simulink subsystem "PvtSubSys_LSM"  (R2020b)
settings: Solver=VariableStepAuto  StartTime=0.0  StopTime=10.0  RelTol=1e-3
values from neighbouring files (symbols this model uses):
  P_LSM_ALC_Enable = 0.0    [LSM_Parameter.sldd]
  P_LSM_DOP_C0_EN_Limit = 0.8    [LSM_Parameter.sldd]
  P_LSM_DOP_C0_out_Limit = 2.0    [LSM_Parameter.sldd]
  P_LSM_DOP_C1_EN_Limit : value not decoded    [LSM_Parameter.sldd]
  P_LSM_DOP_C1_out_Limit : value not decoded    [LSM_Parameter.sldd]
  P_LSM_DOP_C1AndC2_Lim_X : value not decoded    [LSM_Parameter.sldd]
  P_LSM_DOP_C2_EN_Limit : value not decoded    [LSM_Parameter.sldd]
  P_LSM_DOP_C2_out_Limit : value not decoded    [LSM_Parameter.sldd]
  P_LSM_DOP_In_Pre2Dop_Dis = 1.0    [LSM_Parameter.sldd]
  P_LSM_DOP_Out_Pre2Dop_Dis = 2.0    [LSM_Parameter.sldd]
  P_LSM_DOP_PreDis_X : value not decoded    [LSM_Parameter.sldd]
  P_LSM_DOP_PreDis_Y : value not decoded    [LSM_Parameter.sldd]
  P_LSM_DOPValid_CheckTime = 0.06    [LSM_Parameter.sldd]
  P_LSM_DoubleLine_Curr2Cent_Dislimit = 0.5    [LSM_Parameter.sldd]
  P_LSM_DoubleLine_Dop2Cent_Dislimit = 0.5    [LSM_Parameter.sldd]
  P_LSM_DoubleLine_DOPOut_C1 : value not decoded    [LSM_Parameter.sldd]
  P_LSM_DoubleLine_Pre2Cent_Dislimit = 1.0    [LSM_Parameter.sldd]
  P_LSM_IFV2CenterAxis = 0.0    [LSM_Parameter.sldd]
  P_LSM_IFV2RearAxis = 0.0    [LSM_Parameter.sldd]
  P_LSM_LineSTD_Limit = 0.15    [LSM_Parameter.sldd]
  P_LSM_NOH_Switch = 0.0    [LSM_Parameter.sldd]
  P_LSM_Pre_t = 0.0    [LSM_Parameter.sldd]
  P_LSM_SingleLine_Cent2Edge_Dislimit = 100.0    [LSM_Parameter.sldd]
  P_LSM_SingleLine_Curr2Cent_Dislimit = 0.2    [LSM_Parameter.sldd]
  P_LSM_SingleLine_Dop2Cent_Dislimit = 0.2    [LSM_Parameter.sldd]
  P_LSM_SingleLine_DOPOut_C1 : value not decoded    [LSM_Parameter.sldd]
  P_LSM_SingleLine_Pre2Cent_Dislimit = 0.5    [LSM_Parameter.sldd]
undefined symbols (not defined in the file or in its folder): P_LSM_LineWijCal_C12, P_LSM_LineWijCal_C13, P_LSM_PosLineLcFac
libraries: simulink x92, TrueDurationTime x2
(part 8 of 9)

== matlab function PvtSubSys_LSM/Subsystem/TargetLineCalc_20ms/TargetLineCalc/VehStation ==
  data: VisLineConf input uint8; LeftMostLane output boolean; VisLineA0 input single; VisLineType input uint8; VisEdgeConf input uint8; VisEdgeA0 input single; RightMostLane output boolean; VisLineColor input
function [LeftMostLane,RightMostLane] = fcn(VisLineConf,VisLineA0,VisLineType,VisEdgeConf,VisEdgeA0,VisLineColor)
LeftMostLane = false;
RightMostLane = false;
% SingleLane = false;
if (VisLineConf(2)>0&&VisEdgeConf(1)>0&&VisLineType(1)==1&&abs(VisLineA0(2)-VisEdgeA0(1))<5)||VisLineColor(1)==2
    LeftMostLane = true;
elseif (VisLineConf(3)>0&&VisEdgeConf(2)>0&&VisLineType(2)==1&&abs(VisLineA0(3)-VisEdgeA0(2))<5)||VisLineColor(2)==2
    RightMostLane = true;
end

== matlab function PvtSubSys_LSM/Subsystem/TargetLineCalc_20ms/TargetLineCalc/VisLineFilter1 ==
  data: tCycle input single size=1; vRef input; OTLineValid input boolean size=1; aOTL input single size=1; bOTL input single size=1; cOTL input single size=1; dOTL input single size=1; R input single size=1; LineUpdate input boolean size=1; dDeltaX input single size=1; dDeltaY input single size=1; CosOfPsi input single size=1; SinOfPsi input single size=1; LineValidK1 input boolean size=1; A3K1 input single size=1; A2K1 input single size=1; A1K1 input single size=1; A0K1 input single size=1; RangeK1 input single size=1; tLostK1 input single size=1; LineValid output boolean size=1; A3 output single size=1; A2 output single size=1; A1 output single size=1; A0 output single size=1; Range output single size=1; tLost output single size=1
function [LineValid,A3,A2,A1,A0,Range,tLost] = ...
    VisFilter(tCycle,vRef,OTLineValid,aOTL,bOTL,cOTL,dOTL,R,LineUpdate,...
    dDeltaX,dDeltaY,CosOfPsi,SinOfPsi,...
    LineValidK1,A3K1,A2K1,A1K1,A0K1,RangeK1,tLostK1)

if (OTLineValid==true)&&(LineUpdate==true)
    LineValid = true;
    A3 = aOTL;
    A2 = bOTL;
    A1 = cOTL;
    A0 = dOTL;
    Range = R;
%     if Range<RangeK1
%         Range = RangeK1 - vRef*tCycle;
%     end
    tLost = single(0);
else
    tLost = min(tLostK1 + tCycle,single(10));
    if (LineValidK1==true)&&(tLost<1)&&vRef>1.8
        xi = [0;0.25*RangeK1;0.5*RangeK1;RangeK1];
        yi = A3K1*xi.^3 + A2K1*xi.^2 + A1K1*xi + A0K1;
        t_dx = xi-dDeltaX;
        t_dy = yi-dDeltaY;
        TmpX = t_dx*CosOfPsi+t_dy*SinOfPsi;
        TmpY = -t_dx*SinOfPsi+t_dy*CosOfPsi;
        [A3,A2,A1,A0] = pl(TmpX,TmpY);
        LineValid = true;
        Range = RangeK1 - vRef*tCycle;
        if Range<1
            LineValid = false;
        end
    elseif LineValidK1==true&&vRef<=1.8
         xi = [0;0.25*RangeK1;0.5*RangeK1;RangeK1];
        yi = A3K1*xi.^3 + A2K1*xi.^2 + A1K1*xi + A0K1;
        t_dx = xi-dDeltaX;
        t_dy = yi-dDeltaY;
        TmpX = t_dx*CosOfPsi+t_dy*SinOfPsi;
        TmpY = -t_dx*SinOfPsi+t_dy*CosOfPsi;
        [A3,A2,A1,A0] = pl(TmpX,TmpY);
        LineValid = true;
        Range = max(single(5),RangeK1);
    else
        LineValid = false;
        A3 = single(0);
        A2 = single(0);
        A1 = single(0);
        A0 = single(0);
        Range = single(0);
    end
end

== matlab function PvtSubSys_LSM/Subsystem/TargetLineCalc_20ms/TargetLineCalc/VisLineFilter2 ==
  data: tF input single size=1; DevValid output boolean size=4; DevAngle output single size=4; DevDis output single size=4; tCycle input single size=1; VisLineConf input uint8 size=4; VisLineReliable input single; a3 input single size=4; a2 input single size=4; a1 input single size=4; a0 input single size=4; R input single size=4; LineUpdate input boolean size=1; dDeltaX input single size=1; dDeltaY input single size=1; CosOfPsi input single size=1; SinOfPsi input single size=1; vRef input single size=1; Lowlimit input single; RoadWidth input single size=1; LeftLineChange input boolean size=1; RightLineChange input boolean size=1; LH1Wij input single; LH2Wij input single; LineConfK1 input uint8 size=4; LineReliableK1 input single; A3K1 input single size=4; A2K1 input single size=4; A1K1 input single size=4; A0K1 input single size=4; RangeK1 input single size=4; tLostK1 input single size=4; LineConf output uint8 size=4; LineReliable output single; A3 output single size=4; A2 output single size=4; A1 output single size=4; A0 output single size=4; Range output single size=4; tLost output single size=4; Avail_timeK1 input single; Avail_disK1 input single; Avail_time output single; Avail_dis output single; fix_timeK1 input; FaultK1 input; fix_time output; Fault output
    function [DevValid,DevAngle,DevDis,LineConf,LineReliable,A3,A2,A1,A0,Range,tLost,Avail_time,Avail_dis,fix_time,Fault] = ...
    VisFilter(tF,tCycle,VisLineConf,VisLineReliable,a3,a2,a1,a0,R,LineUpdate,...
    dDeltaX,dDeltaY,CosOfPsi,SinOfPsi,vRef,Lowlimit,RoadWidth,LeftLineChange,RightLineChange,LH1Wij,LH2Wij,...
    LineConfK1, LineReliableK1,A3K1,A2K1,A1K1,A0K1,RangeK1,tLostK1,Avail_timeK1,Avail_disK1,fix_timeK1,FaultK1)

LineConf = uint8(zeros(4,1));
LineReliable = single(zeros(4,1));
A3 = single(zeros(4,1));
A2 = single(zeros(4,1));
A1 = single(zeros(4,1));
A0 = single(zeros(4,1));
Range = single(zeros(4,1));
tLost = single(zeros(4,1));

Line_std = single(zeros(4,1));
Avail_time = Avail_timeK1;
Avail_dis = Avail_disK1;
fix_time = fix_timeK1;
Fault = FaultK1;

DevValid = false(4,1);
DevAngle = single(zeros(4,1));
DevDis = single(zeros(4,1));

for i=1:4
    if  (LineUpdate==true)&&(VisLineConf(i)>0)&&VisLineReliable(i)>0.01  
        LineConf(i) = VisLineConf(i);
        LineReliable(i) = VisLineReliable(i);
        A3(i) = a3(i);
        A2(i) = a2(i);
        A1(i) = a1(i);
        A0(i) = a0(i);
        Range(i) = R(i);
        if Range(i)<RangeK1(i)
            Range(i) = RangeK1(i) - vRef*tCycle;
        end
        tLost(i) = single(0);
        
        if LineConfK1(i)>0
            DevValid(i) = true;
            t_Dist = max(single(15),vRef*1.8);
            xi = [0.05*t_Dist;0.3*t_Dist;0.6*t_Dist;t_Dist];
            yi = A3K1(i)*xi.^3 + A2K1(i)*xi.^2 + A1K1(i)*xi + A0K1(i);
            t_dx = xi-dDeltaX;
            t_dy = yi-dDeltaY;
            TmpX = t_dx*CosOfPsi+t_dy*SinOfPsi;
            TmpY = -t_dx*SinOfPsi+t_dy*CosOfPsi;
            [t3,t2,t1,t0] = pl(TmpX,TmpY);
            
            DevAngle(i) = 57.3*(atan(A1(i)) - atan(t1));
            DevDis(i) = (A0(i) - t0)/sqrt(A1(i)^2 + single(1));
            
            if (abs(DevAngle(i))<3)&&(abs(DevDis(i))<0.06)
                tFilter = 0.05/tF;
                A3(i) = tFilter*(A3(i) - t3) + t3;
                A2(i) = tFilter*(A2(i) - t2) + t2;
                A1(i) = tFilter*(A1(i) - t1) + t1;
                A0(i) = tFilter*(A0(i) - t0) + t0;
            end
        end
    else
        tLost(i) = min(tLostK1(i) + tCycle,single(10));
        if (LineConfK1(i)>0)&&(tLost(i)<0.5)&&vRef>1.8
            xi = [0.5*vRef;(0.5*vRef+0.25*RangeK1(i));(0.5*vRef+0.5*RangeK1(i));(0.5*vRef+RangeK1(i))];
            yi = A3K1(i)*xi.^3 + A2K1(i)*xi.^2 + A1K1(i)*xi + A0K1(i);
            t_dx = xi-dDeltaX;
            t_dy = yi-dDeltaY;
            TmpX = t_dx*CosOfPsi+t_dy*SinOfPsi;
            TmpY = -t_dx*SinOfPsi+t_dy*CosOfPsi;
            [A3(i),A2(i),A1(i),A0(i)] = pl(TmpX,TmpY);
            LineConf(i) = LineConfK1(i);
            LineReliable(i) = LineReliableK1(i);
            Range(i) = RangeK1(i) - 0.5*vRef*tCycle;
            if Range(i)<5
                LineConf(i) = uint8(0);
            end
        elseif (LineConfK1(i)>0)&&vRef<=1.8
            xi = [0.5*vRef;(0.5*vRef+0.25*RangeK1(i));(0.5*vRef+0.5*RangeK1(i));(0.5*vRef+RangeK1(i))];
            yi = A3K1(i)*xi.^3 + A2K1(i)*xi.^2 + A1K1(i)*xi + A0K1(i);
            t_dx = xi-dDeltaX;
            t_dy = yi-dDeltaY;
            TmpX = t_dx*CosOfPsi+t_dy*SinOfPsi;
            TmpY = -t_dx*SinOfPsi+t_dy*CosOfPsi;
            [A3(i),A2(i),A1(i),A0(i)] = pl(TmpX,TmpY);
            LineConf(i) = LineConfK1(i);
            LineReliable(i) = LineReliableK1(i);
            Range(i) = max(5,RangeK1(i));
        end
    end
end
%%  车道线校验
if LeftLineChange
    Avail_time = [single(0);Avail_timeK1(1)+tCycle;Avail_timeK1(2)+tCycle;Avail_timeK1(3)+tCycle];
    Avail_dis = [single(0);Avail_disK1(1)+tCycle*vRef;Avail_disK1(2)+tCycle*vRef;Avail_disK1(3)+tCycle*vRef];  
elseif RightLineChange
    Avail_time = [Avail_timeK1(2)+tCycle;Avail_timeK1(3)+tCycle;Avail_timeK1(4)+tCycle;single(0)];
    Avail_dis = [Avail_disK1(2)+tCycle*vRef;Avail_disK1(3)+tCycle*vRef;Avail_disK1(4)+tCycle*vRef;single(0)];
else
    for i = 1:4
        if  LineConf(i)>0
            t_Dist = max(single(15),5*vRef);
            xi = [0.05*t_Dist;0.6*t_Dist;0.8*t_Dist;t_Dist];
            yi = A3K1(i)*xi.^3 + A2K1(i)*xi.^2 + A1K1(i)*xi + A0K1(i);
            t_dx = xi-dDeltaX;
            y = A3(i)*t_dx.^3+A2(i)*t_dx.^2+A1(i)*t_dx+A0(i);
            Error = y - yi;
            Line_std(i) = std(Error);
            if Line_std(i)<Lowlimit
                Avail_time(i) = Avail_timeK1(i)+tCycle;
                Avail_dis(i) = Avail_disK1(i)+tCycle*vRef;
            else
                Avail_time(i) = single(0);
                Avail_dis(i) = single(0);
            end
%             if Avail_time(i)>6&&Avail_dis(i)>60
%                 Fault(i) = false;
%             end
%             if Fault(i)==true
%                 fix_time(i) = fix_timeK1(i)+tCycle;
%                 xi = [0.5*vRef;(0.5*vRef+0.25*RangeK1(i));(0.5*vRef+0.5*RangeK1(i));(0.5*vRef+RangeK1(i))];
%                 yi = A3K1(i)*xi.^3 + A2K1(i)*xi.^2 + A1K1(i)*xi + A0K1(i);
%                 t_dx = xi-dDeltaX;
%                 t_dy = yi-dDeltaY;
%                 TmpX = t_dx*CosOfPsi+t_dy*SinOfPsi;
%                 TmpY = -t_dx*SinOfPsi+t_dy*CosOfPsi;
%                 [A3(i),A2(i),A1(i),A0(i)] = pl(TmpX,TmpY);
%                 LineConf(i) = LineConfK1(i);
%                 LineReliable(i) = LineReliableK1(i);
%                 Range(i) = RangeK1(i) - 0.5*vRef*tCycle;
%                 if Range(i)<10||fix_time(i)>2
%                     LineConf(i) = uint8(0);
%                 end
%             else
%                 fix_time(i) = single(0);
%             end
        elseif LineConf(i)==0
            Avail_time(i) = single(0);
            Avail_dis(i) = single(0);
        end
    end
end
Avail_time = min(Avail_time,single(10));
Avail_dis = min(Avail_dis,single(100));

%%   
%    When occur left-line crossing,if L2 lost,the above line offset
%    algorithm may calculate a new L2 line,but now the new L2 line have
%    became L3 line ,so it lead to L2 line and L3 line are the same
if (LeftLineChange||RightLineChange) && VisLineConf(2)==0                       
    A3(2) = A3(3);
    A2(2) = A2(3);
    A1(2) = A1(3);
    A0(2) = A0(3)+RoadWidth*sqrt(1+A1(3)*A1(3));
    LineConf(2) = LineConf(3);
    LineReliable(2) = LineReliable(3);
    Range(2) = Range(3);
elseif  (LeftLineChange||RightLineChange) && VisLineConf(3)==0
    A3(3) = A3(2);
    A2(3) = A2(2);
    A1(3) = A1(2);
    A0(3) = A0(2)-RoadWidth*sqrt(1+A1(2)*A1(2));
    LineConf(3) = LineConf(2);
    LineReliable(3) = LineReliable(2);
    Range(3) = Range(2);
end

== matlab function PvtSubSys_LSM/Subsystem/TargetLineCalc_20ms/TargetLineCalc/VisLineFilter4 ==
  data: EdgeConf output uint8 size=2; EdgeReliable output single; EdgeA3 output single size=2; EdgeA2 output single size=2; EdgeA1 output single size=2; EdgeA0 output single size=2; tCycle input single size=1; VisEdgeConf input uint8 size=2; VisEdgeReliable input single; a3 input single size=2; a2 input single size=2; a1 input single size=2; a0 input single size=2; R input single size=2; LineUpdate input boolean size=1; dDeltaX input single size=1; dDeltaY input single size=1; CosOfPsi input single size=1; SinOfPsi input single size=1; vRef input single size=1; EdgeConfK1 input uint8 size=2; EdgeReliableK1 input single; EdgeA3K1 input single size=2; EdgeA2K1 input single size=2; EdgeA1K1 input single size=2; EdgeA0K1 input single size=2; EdgeRangeK1 input single size=2; EdgetLostK1 input single size=2; EdgeRange output single size=2; EdgetLost output single size=2; Avail_timeK1 input single; Avail_disK1 input single; Avail_time output single; Avail_dis output single
function [EdgeConf,EdgeReliable,EdgeA3,EdgeA2,EdgeA1,EdgeA0,EdgeRange,EdgetLost,Avail_time,Avail_dis] = ...
    VisFilter(tCycle,VisEdgeConf,VisEdgeReliable,a3,a2,a1,a0,R,LineUpdate,...
    dDeltaX,dDeltaY,CosOfPsi,SinOfPsi,vRef,EdgeConfK1,EdgeReliableK1,EdgeA3K1,...
    EdgeA2K1,EdgeA1K1,EdgeA0K1,EdgeRangeK1,EdgetLostK1,Avail_timeK1,Avail_disK1)

EdgeConf = uint8(zeros(2,1));
EdgeReliable = single(zeros(2,1));
EdgeA3 = single(zeros(2,1));
EdgeA2 = single(zeros(2,1));
EdgeA1 = single(zeros(2,1));
EdgeA0 = single(zeros(2,1));
EdgeRange = single(zeros(2,1));
EdgetLost = single(zeros(2,1));
Line_std = single(zeros(2,1));
Avail_time = Avail_timeK1;
Avail_dis = Avail_disK1;

for i=1:2
    if (VisEdgeConf(i)>0)&&(LineUpdate==true)
        EdgeConf(i) = VisEdgeConf(i);
        EdgeReliable(i) = VisEdgeReliable(i);
        EdgeA3(i) = a3(i);
        EdgeA2(i) = a2(i);
        EdgeA1(i) = a1(i);
        EdgeA0(i) = a0(i);
        EdgeRange(i) = R(i);
        EdgetLost(i) = single(0);
    else
        EdgetLost(i) = min(EdgetLostK1(i) + tCycle,single(10));
        if (EdgeConfK1(i)>0)&&(EdgetLost(i)<0.3)
            xi = [0.5*vRef;(0.5*vRef+0.25*EdgeRangeK1(i));(0.5*vRef+0.5*EdgeRangeK1(i));(0.5*vRef+EdgeRangeK1(i))];
            yi = EdgeA3K1(i)*xi.^3 + EdgeA2K1(i)*xi.^2 + EdgeA1K1(i)*xi + EdgeA0K1(i);
            t_dx = xi-dDeltaX;
            t_dy = yi-dDeltaY;
            TmpX = t_dx*CosOfPsi+t_dy*SinOfPsi;
            TmpY = -t_dx*SinOfPsi+t_dy*CosOfPsi;
            [EdgeA3(i),EdgeA2(i),EdgeA1(i),EdgeA0(i)] = pl(TmpX,TmpY);
            EdgeConf(i) = EdgeConfK1(i);
            EdgeReliable(i) = EdgeReliableK1(i);
            EdgeRange(i) = EdgeRangeK1(i) - 0.25*vRef*tCycle;
            
            if EdgeRange(i)<5
                EdgeConf(i) = uint8(0);
            end
            
        else
            EdgeConf(i) = uint8(0);
            EdgeReliable(i) = single(0);
            EdgeA3(i) = single(0);
            EdgeA2(i) = single(0);
            EdgeA1(i) = single(0);
            EdgeA0(i) = single(0);
            EdgeRange(i) = single(0);
        end
    end
end
%%  边界线校验
for i = 1:2
    if EdgeConf(i)>0
        t_Dist = max(single(15),3*vRef);
        xi = [0.05*t_Dist;0.6*t_Dist;0.8*t_Dist;t_Dist];
        yi = EdgeA3K1(i)*xi.^3 + EdgeA2K1(i)*xi.^2 + EdgeA1K1(i)*xi + EdgeA0K1(i);
        t_dx = xi-dDeltaX;
        y = EdgeA3(i)*t_dx.^3+EdgeA2(i)*t_dx.^2+EdgeA1(i)*t_dx+EdgeA0(i);
        Error = y - yi;
        Line_std(i) = std(Error);
        if Line_std(i)<0.15
            Avail_time(i) = Avail_timeK1(i)+tCycle;
            Avail_dis(i) = Avail_disK1(i)+tCycle*vRef;
        else
            Avail_time(i) = single(0);
            Avail_dis(i) = single(0);
        end
    elseif EdgeConf(i)==0
        Avail_time(i) = single(0);
        Avail_dis(i) = single(0);
    end
end

== matlab function PvtSubSys_LSM/Subsystem/TargetLineCalc_20ms/TargetLineCalc/YBranchRi ==
  data: LineUpdate input boolean size=1; RightOffset_b input boolean size=1; vRef input single size=1; RoadWidth input single size=1; A3 input single size=4; A2 input single size=4; A1 input single size=4; A0 input single size=4; Conf input uint8 size=4; Reliable input; DistK1 input single size=1; YBranch_b output boolean size=1; YBranchRi_b output boolean size=1; Dist output single size=1; DistRiK1 input single size=1; DistRi output single size=1
function [YBranch_b,YBranchRi_b,Dist,DistRi] =...
    fcn(LineUpdate,RightOffset_b,vRef,RoadWidth,A3,A2,A1,A0,Conf,Reliable,DistK1,DistRiK1)
%%  判断本车道40米处是否边宽变窄，或者右侧出现分叉车道
Dist = max(DistK1 - 0.02*vRef,single(0));
DistRi = max(DistRiK1 - 0.02*vRef,single(0));
if RightOffset_b
    Dist = DistRi;
    DistRi = single(0);
end
LConf = uint8(0);
RConf = uint8(0);
RRConf = uint8(0);
LA3 = A3(2);
LA2 = A2(2);
LA1 = A1(2); 
LA0 = A0(2);
if Reliable(2)>=0.9
LConf = Conf(2);
end

RA3 = A3(3);
RA2 = A2(3);
RA1 = A1(3); 
RA0 = A0(3);
if Reliable(3)>=0.9
RConf = Conf(3);
end

RRA3 = A3(4);
RRA2 = A2(4);
RRA1 = A1(4); 
RRA0 = A0(4);
if Reliable(4)>=0.9
RRConf = Conf(4);
end

if (LConf>0)&&(RConf>0)&&(LineUpdate)&&abs(LA2)<0.0005&&abs(RA2)<0.0005
    dy0 = (LA0 - RA0)/sqrt(LA1^2 +single(1));
    dy40L = 64000*LA3 + 1600*LA2 + 40*LA1 + LA0;
    dy40R = 64000*RA3 + 1600*RA2 + 40*RA1 + RA0;
    K40 = 3*LA3*1600 + 2*LA2*40 + LA1;
    dy40 = (dy40L - dy40R)/sqrt(K40^2 +single(1));
    if (dy0 - dy40<-0.5)&&(RoadWidth>2.5)&&(RoadWidth<4.2)
        Dist = single(20);
    end
end

if Dist>0
    YBranch_b = true;
else
    YBranch_b = false;
end

if (RConf>0)&&(RRConf>0)&&(LineUpdate)
    dy0 = (RA0 - RRA0)/sqrt(RA1^2 + single(1));
    dy40L = 64000*RA3 + 1600*RA2 + 40*RA1 + RA0;
    dy40R = 64000*RRA3 + 1600*RRA2 + 40*RRA1 + RRA0;
    K40 = 3*RA3*1600 + 2*RA2*40 + RA1;
    dy40 = (dy40L - dy40R)/sqrt(K40^2 + single(1));
    if (vRef>15)&&(abs(dy0 - dy40)>1.0)&&(RoadWidth>2.5)&&(RoadWidth<4.2)
        DistRi = single(20);
    end
end

if DistRi>0
    YBranchRi_b = true;
else
    YBranchRi_b = false;
end

== matlab function PvtSubSys_LSM/Subsystem/TargetLineCalc_20ms/TargetLineCalc/MATLAB Function ==
  data: Cur_avail input; MrcStopLane output; Cur_LaneType input; Right_avail input
function MrcStopLane = fcn(Cur_avail,Cur_LaneType,Right_avail)
MrcStopLane = uint8(0);
if (Cur_avail>0&&Cur_LaneType==5)||(Cur_avail>0&&Cur_LaneType~=5&&Right_avail==0)
    MrcStopLane = uint8(1);
end

== matlab function PvtSubSys_LSM/Subsystem/TargetLineCalc_20ms/TargetLineCalc/MATLAB Function2 ==
  data: LH1Wij input; LH2Wij input; LH1_Valid output; LH2_Valid output; Wij_state output; kap input; preDis input; VisLineA3 input; VisLineA2 input; VisLineA1 input; VisLineA0 input
function [LH1_Valid,LH2_Valid,Wij_state] = fcn(LH1Wij,LH2Wij,...
    kap,preDis,VisLineA3,VisLineA2,VisLineA1,VisLineA0)

LH1_Valid = false;
LH2_Valid = false;
Wij_state = uint8(0);

dy_pre = 0.5*kap*preDis^2;
Curature2_pre = VisLineA1(2) + 2*VisLineA2(2)*preDis + 3*VisLineA3(2)*(preDis^2);
Curature3_pre = VisLineA1(3) + 2*VisLineA2(3)*preDis + 3*VisLineA3(3)*(preDis^2);
dy2 = (VisLineA0(2) + VisLineA1(2)*preDis + VisLineA2(2)*(preDis^2) + VisLineA3(2)*(preDis^3) - dy_pre)/sqrt(Curature2_pre^2+single(1));
dy3 = (VisLineA0(3) + VisLineA1(3)*preDis + VisLineA2(3)*(preDis^2) + VisLineA3(3)*(preDis^3) - dy_pre)/sqrt(Curature3_pre^2+single(1));
RoadWidth_Cur = VisLineA0(2)-VisLineA0(3);

if LH1Wij >= 0.3 && LH2Wij >= 0.3  %置信度都比较高
%     if LeftLightReq
%        LH1_Valid = true;
%        Wij_state = uint8(1);
%     elseif RightLightReq  %开启右转向
%         LH2_Valid = true;
%         Wij_state = uint8(2);
%     elseif StubValid>0 && StubStartDis<60 && (Direction==3 || Direction==1)  % 导航向左
%                 LH1_Valid = true;
%                 Wij_state = uint8(3);
%     elseif StubValid>0 && StubStartDis<60 && (Direction==4 || Direction==2)  % 导航向右
%                 LH2_Valid = true;
%                 Wij_state = uint8(4);
    
    if RoadWidth_Cur-(dy2-dy3)>0.5  || dy2-dy3-RoadWidth_Cur>0.5 ||...
            abs(VisLineA0(2) - VisLineA0(3))>4.2 ||...
            abs(VisLineA0(2) - VisLineA0(3))<2.6     %没方向，有分叉或过宽、过窄
        if LH1Wij >= LH2Wij
            LH1_Valid = true;
            Wij_state = uint8(3);
        else
            LH2_Valid = true;
            Wij_state = uint8(4);
        end
    else  %没方向，没分叉
        LH1_Valid = true;
        LH2_Valid = true;
        Wij_state = uint8(5);
    end
    
elseif LH1Wij >= 0.3 
    LH1_Valid = true;
    Wij_state = uint8(1);
elseif LH2Wij >= 0.3
    LH2_Valid = true;
    Wij_state = uint8(2);
end

== matlab function PvtSubSys_LSM/Subsystem/TargetLineCalc_20ms/TargetLineCalc/MATLAB Function3 ==
  data: LH1_Valid input; LH2_Valid input; CentLineValid output; VisLineA3 input; VisLineA2 input; VisLineA1 input; VisLineA0 input; VisLineR input; RoadWidth input; CentLineC3 output; CentLineC2 output; CentLineC1 output; CentLineC0 output; CentLineRange output; CentLineReliable output; Line_State output; LH1Wij input; LH2Wij input
function [CentLineValid,CentLineC3,CentLineC2,CentLineC1,CentLineC0,CentLineRange,CentLineReliable,Line_State] = ...
    VisFilter(LH1_Valid,LH2_Valid,...
    VisLineA3,VisLineA2,VisLineA1,VisLineA0,VisLineR,RoadWidth,LH1Wij,LH2Wij)

CentLineValid = false;
CentLineC0 = single(0);
CentLineC1 = single(0);
CentLineC2 = single(0);
CentLineC3 = single(0);
CentLineRange = single(0);
CentLineReliable = single(0);
Line_State = uint8(0);

if (LH1_Valid) && (LH2_Valid)
    Range_Error = VisLineR(2) - VisLineR(3);
    LH1_Offset = single(0.5);
    LH2_Offset = single(0.5);
    if Range_Error>10 || Range_Error<-10
        LH1_Offset = 0.5+min(0.5,Range_Error*0.01);
        LH2_Offset = 1-LH1_Offset;
    end
    CentLineValid = true;
    CentLineC0 = 0.5*(VisLineA0(2) + VisLineA0(3));
    CentLineC1 = LH1_Offset*VisLineA1(2) + LH2_Offset*VisLineA1(3);
    CentLineC2 = LH1_Offset*VisLineA2(2) + LH2_Offset*VisLineA2(3);
    CentLineC3 = LH1_Offset*VisLineA3(2) + LH2_Offset*VisLineA3(3);
    CentLineRange = max(VisLineR(2),VisLineR(3));
    CentLineReliable = 0.5*(LH1Wij+LH2Wij);
    Line_State = uint8(1);
elseif LH1_Valid
    CentLineValid = true;
    CentLineC0 = VisLineA0(2)-0.5*RoadWidth*sqrt(1+VisLineA1(2)*VisLineA1(2));
    CentLineC1 = VisLineA1(2);
    CentLineC2 = VisLineA2(2);
    CentLineC3 = VisLineA3(2);
    CentLineRange = VisLineR(2);
    CentLineReliable = LH1Wij;
    Line_State = uint8(2);
elseif LH2_Valid
    CentLineValid = true;
    CentLineC0 = VisLineA0(3)+0.5*RoadWidth*sqrt(1+VisLineA1(3)*VisLineA1(3));
    CentLineC1 = VisLineA1(3);
    CentLineC2 = VisLineA2(3);
    CentLineC3 = VisLineA3(3);
    CentLineRange = VisLineR(3);
    CentLineReliable = LH2Wij;
    Line_State = uint8(3);
end

== matlab function PvtSubSys_LSM/Subsystem/TargetLineCalc_20ms/TargetLineCalc/MATLAB Function4 ==
  data: LH1Wij input; LH2Wij input; LH1_Valid input; LH2_Valid input; CentLineValid output; VisLineConf input; VisLineA3 input; VisLineA2 input; VisLineA1 input; VisLineA0 input; VisLineR input; RoadWidth input; CentLineC3 output; CentLineC2 output; CentLineC1 output; CentLineC0 output; CentLineRange output; CentLineReliable output; LeftLineValid output; LeftLineC3 output; LeftLineC2 output; LeftLineC1 output; LeftLineC0 output; LeftLineRange output; LeftLineReliable output; LeftLaneAvail output; RightLineValid output; RightLineC3 output; RightLineC2 output; RightLineC1 output; RightLineC0 output; RightLineRange output; RightLineReliable output; RightLaneAvail output; Line_State output; preDis input
function [CentLineValid,CentLineC3,CentLineC2,CentLineC1,CentLineC0,CentLineRange,CentLineReliable,...
    LeftLineValid,LeftLineC3,LeftLineC2,LeftLineC1,LeftLineC0,LeftLineRange,LeftLineReliable,LeftLaneAvail,...
    RightLineValid,RightLineC3,RightLineC2,RightLineC1,RightLineC0,RightLineRange,RightLineReliable,RightLaneAvail,...
    Line_State] = ...
    VisFilter(LH1Wij,LH2Wij,LH1_Valid,LH2_Valid,...
    VisLineConf,VisLineA3,VisLineA2,VisLineA1,VisLineA0,VisLineR,RoadWidth,preDis)

CentLineValid = false;
CentLineC0 = single(0);
CentLineC1 = single(0);
CentLineC2 = single(0);
CentLineC3 = single(0);
CentLineRange = single(0);
CentLineReliable = single(0);
Line_State = uint8(0);

if (LH1_Valid) && (LH2_Valid)
    Range_Error = VisLineR(2) - VisLineR(3);
    LH1_Offset = single(0.5);
    LH2_Offset = single(0.5);
    if Range_Error>10 || Range_Error<-10
        LH1_Offset = 0.5+min(0.5,Range_Error*0.01);
        LH2_Offset = 1-LH1_Offset;
    end
    CentLineValid = true;
    CentLineC0 = 0.5*(VisLineA0(2) + VisLineA0(3));
    CentLineC1 = LH1_Offset*VisLineA1(2) + LH2_Offset*VisLineA1(3);
    CentLineC2 = LH1_Offset*VisLineA2(2) + LH2_Offset*VisLineA2(3);
    CentLineC3 = LH1_Offset*VisLineA3(2) + LH2_Offset*VisLineA3(3);
    CentLineRange = max(VisLineR(2),VisLineR(3));
    CentLineReliable = 0.5*(LH1Wij+LH2Wij);
    Line_State = uint8(3);
elseif LH1_Valid
    CentLineValid = true;
    CentLineC0 = VisLineA0(2)-0.5*RoadWidth*sqrt(1+VisLineA1(2)*VisLineA1(2));
    CentLineC1 = VisLineA1(2);
    CentLineC2 = VisLineA2(2);
    CentLineC3 = VisLineA3(2);
    CentLineRange = VisLineR(2);
    CentLineReliable = LH1Wij;
    Line_State = uint8(1);
elseif LH2_Valid
    CentLineValid = true;
    CentLineC0 = VisLineA0(3)+0.5*RoadWidth*sqrt(1+VisLineA1(3)*VisLineA1(3));
    CentLineC1 = VisLineA1(3);
    CentLineC2 = VisLineA2(3);
    CentLineC3 = VisLineA3(3);
    CentLineRange = VisLineR(3);
    CentLineReliable = LH2Wij;
    Line_State = uint8(2);
end

if LH1Wij>=0.3
    LeftLineValid = true;
    LeftLineC0 = VisLineA0(2) + 0.5*RoadWidth*sqrt(1+VisLineA1(2)*VisLineA1(2));
    LeftLineC1 = VisLineA1(2);
    LeftLineC2 = VisLineA2(2);
    LeftLineC3 = VisLineA3(2);
    LeftLineRange = VisLineR(2);
    LeftLineReliable = LH1Wij;
    t1 = VisLineA0(1)+VisLineA1(1)*preDis+VisLineA2(1)*preDis^2+VisLineA3(1)*preDis^3;
    t2 = VisLineA0(2)+VisLineA1(2)*preDis+VisLineA2(2)*preDis^2+VisLineA3(2)*preDis^3; 
    if (VisLineConf(1)>0)&&...
            ((VisLineA0(1)-VisLineA0(2))>3)&&...
            ((VisLineA0(1)-VisLineA0(2))<5.5)&&...
            ((t1 - t2)>3)
        LeftLaneAvail = true;
    else
        LeftLaneAvail = false;
    end
else
    LeftLineValid = false;
    LeftLineC0 = single(0);
    LeftLineC1 = single(0);
    LeftLineC2 = single(0);
    LeftLineC3 = single(0);
    LeftLineRange = single(0);
    LeftLineReliable = single(0);
    LeftLaneAvail = false;
end

if LH2Wij>=0.3
    RightLineValid = true;
    RightLineC0 = VisLineA0(3) - 0.5*RoadWidth*sqrt(1+VisLineA1(3)*VisLineA1(3));
    RightLineC1 = VisLineA1(3);
    RightLineC2 = VisLineA2(3);
    RightLineC3 = VisLineA3(3);
    RightLineRange = VisLineR(3);
    RightLineReliable = LH2Wij;
    
    t3 = VisLineA0(3)+VisLineA1(3)*preDis+VisLineA2(3)*preDis^2+VisLineA3(3)*preDis^3;
    t4 = VisLineA0(4)+VisLineA1(4)*preDis+VisLineA2(4)*preDis^2+VisLineA3(4)*preDis^3;

    if (VisLineConf(4)>0)&&...
            ((VisLineA0(3)-VisLineA0(4))>3)&&...
            ((VisLineA0(3)-VisLineA0(4))<5.5)&&...
            ((t3 - t4)>3)

        RightLaneAvail = true;
    else
        RightLaneAvail = false;
    end
else
    RightLineValid = false;
    RightLineC0 = single(0);
    RightLineC1 = single(0);
    RightLineC2 = single(0);
    RightLineC3 = single(0);
    RightLineRange = single(0);
    RightLineReliable = single(0);
    RightLaneAvail = false;
end

== matlab function PvtSubSys_LSM/Subsystem/TargetLineCalc_20ms/TargetLineCalc/Subsystem4/MATLAB Function3 ==
  data: C12 input; Fac1 output single; C13 input; Fac2 output single; Fac3 output single
function [Fac1,Fac2,Fac3]  = fcn(C12,C13)

C21 = 1/C12;
C31 = 1/C13;

C32 = C12/C13;

C23 = C13/C12;



C = [1,   C12,   C13;
    C21,   1,    C23;
    C31,  C32,    1];

Fac1 = 1/(1 + C21 + C31 );
Fac2 = 1/(C12 + 1+ C32 );
Fac3 = 1/(C13 + C23 + 1 );

== matlab function PvtSubSys_LSM/Subsystem/TargetLineCalc_20ms/TargetLineCalc/Subsystem4/MATLAB Function6 ==
  data: kap input; preDis input; CentLineValidK1 input; CentLineC3K1 input; CentLineC2K1 input; CentLineC1K1 input; CentLineC0K1 input; VisLineA3 input; VisLineA2 input; VisLineA1 input; VisLineA0 input; n1 input; n2 input; CosOfPsi input; SinOfPsi input; dDeltaX input; dDeltaY input; d_cur2 output; delta_d2 output; d_cur3 output; delta_d3 output; HWASts input
function [d_cur2,delta_d2,d_cur3,delta_d3] = ...
    fcn( kap,preDis,CentLineValidK1,CentLineC3K1,CentLineC2K1,CentLineC1K1,CentLineC0K1,...
    VisLineA3,VisLineA2,VisLineA1,VisLineA0,n1,n2,...
    CosOfPsi,SinOfPsi,dDeltaX,dDeltaY,HWASts)

xi = [single(1);single(2);single(3);single(4)];
yi = CentLineC3K1*xi.^3 + CentLineC2K1*xi.^2 + CentLineC1K1*xi + CentLineC0K1;
t_dx = xi-dDeltaX;
t_dy = yi-dDeltaY;
TmpX = t_dx*CosOfPsi+t_dy*SinOfPsi;
TmpY = -t_dx*SinOfPsi+t_dy*CosOfPsi;
[t3,t2,t1,t0] = pl(TmpX,TmpY);

if CentLineValidK1
    m1 = n1;
    m2 = n2;
else
    m1 = single(0);
    m2 = single(0);
end


RefA3_2 = t3*m1;
RefA2_2 = t2*m1 + (1-m1)*(0.5*kap);
RefA1_2 = t1*m1;
RefA0_2 = t0*m1;

RefA3_3 = t3*m2;
RefA2_3 = t2*m2 + (1-m2)*(0.5*kap);
RefA1_3 = t1*m2;
RefA0_3 = t0*m2;

y2 = RefA3_2*(preDis^3) + RefA2_2*(preDis^2) + RefA1_2*preDis + RefA0_2;
y3 = RefA3_3*(preDis^3) + RefA2_3*(preDis^2) + RefA1_3*preDis + RefA0_3;

if HWASts == 5 || HWASts == 6
    d_cur2 = abs(VisLineA0(2) - RefA0_2);
    d_cur3 = abs(RefA0_3 - VisLineA0(3));
else
    d_cur2 = VisLineA0(2) - RefA0_2;
    d_cur3 = RefA0_3 - VisLineA0(3);
end


d_pre2 = abs((VisLineA0(2) + VisLineA1(2)*preDis + VisLineA2(2)*(preDis^2) + VisLineA3(2)*(preDis^3)) - y2);  %预瞄点的距离
d_pre3 = abs((VisLineA0(3) + VisLineA1(3)*preDis + VisLineA2(3)*(preDis^2) + VisLineA3(3)*(preDis^3)) - y3);
delta_d2 = abs(d_pre2 - d_cur2);
delta_d3 = abs(d_pre3 - d_cur3);

== matlab function PvtSubSys_LSM/Subsystem/TargetLineCalc_20ms/TargetLineCalc/Subsystem4/MATLAB Function7 ==
  data: dy2_Ran output; L2_R input; dy3_Ran output; L3_R input
function [dy2_Ran,dy3_Ran] = fcn(L2_R,L3_R)
dy2_Ran = L2_R;
dy3_Ran= L3_R;

== matlab function PvtSubSys_LSM/Subsystem/TargetLineCalc_20ms/TargetLineCalc/Subsystem4/MATLAB Function8 ==
  data: VisLineReliable input; dy2_Rel output; dy3_Rel output
function [dy2_Rel,dy3_Rel] = fcn(VisLineReliable)
dy2_Rel = VisLineReliable(2);
dy3_Rel = VisLineReliable(3);

== matlab function PvtSubSys_LSM/Subsystem/TargetLineCalc_20ms/TargetLineCalc/Subsystem5/MATLAB Function3 ==
  data: C12 input; Fac1 output single; C13 input; Fac2 output single; Fac3 output single
function [Fac1,Fac2,Fac3]  = fcn(C12,C13)

C21 = 1/C12;
C31 = 1/C13;

C32 = C12/C13;

C23 = C13/C12;



C = [1,   C12,   C13;
    C21,   1,    C23;
    C31,  C32,    1];

Fac1 = 1/(1 + C21 + C31 );
Fac2 = 1/(C12 + 1+ C32 );
Fac3 = 1/(C13 + C23 + 1 );

== matlab function PvtSubSys_LSM/Subsystem/TargetLineCalc_20ms/TargetLineCalc/Subsystem5/MATLAB Function6 ==
  data: kap input; preDis input; CentLineValidK1 input; CentLineC3K1 input; CentLineC2K1 input; CentLineC1K1 input; CentLineC0K1 input; VisLineA3 input; VisLineA2 input; VisLineA1 input; VisLineA0 input; n1 input; n2 input; CosOfPsi input; SinOfPsi input; dDeltaX input; dDeltaY input; d_cur2 output; delta_d2 output; d_cur3 output; delta_d3 output; HWASts input
function [d_cur2,delta_d2,d_cur3,delta_d3] = ...
    fcn( kap,preDis,CentLineValidK1,CentLineC3K1,CentLineC2K1,CentLineC1K1,CentLineC0K1,...
    VisLineA3,VisLineA2,VisLineA1,VisLineA0,n1,n2,...
    CosOfPsi,SinOfPsi,dDeltaX,dDeltaY, HWASts)

xi = [single(1);single(2);single(3);single(4)];
yi = CentLineC3K1*xi.^3 + CentLineC2K1*xi.^2 + CentLineC1K1*xi + CentLineC0K1;
t_dx = xi-dDeltaX;
t_dy = yi-dDeltaY;
TmpX = t_dx*CosOfPsi+t_dy*SinOfPsi;
TmpY = -t_dx*SinOfPsi+t_dy*CosOfPsi;
[t3,t2,t1,t0] = pl(TmpX,TmpY);

if CentLineValidK1
    m1 = n1;
    m2 = n2;
else
    m1 = single(0);
    m2 = single(0);
end


RefA3_2 = t3*m1;
RefA2_2 = t2*m1 + (1-m1)*(0.5*kap);
RefA1_2 = t1*m1;
RefA0_2 = t0*m1;

RefA3_3 = t3*m2;
RefA2_3 = t2*m2 + (1-m2)*(0.5*kap);
RefA1_3 = t1*m2;
RefA0_3 = t0*m2;

y2 = RefA3_2*(preDis^3) + RefA2_2*(preDis^2) + RefA1_2*preDis + RefA0_2;
y3 = RefA3_3*(preDis^3) + RefA2_3*(preDis^2) + RefA1_3*preDis + RefA0_3;

if HWASts == 5 ||HWASts == 6
    d_cur2 = abs( VisLineA0(2) - RefA0_2);
    d_cur3 = abs(RefA0_3 - VisLineA0(3));
else
    d_cur2 = VisLineA0(2) - RefA0_2;
    d_cur3 = RefA0_3 - VisLineA0(3);
end


d_pre2 = abs((VisLineA0(2) + VisLineA1(2)*preDis + VisLineA2(2)*(preDis^2) + VisLineA3(2)*(preDis^3)) - y2);  %预瞄点的距离
d_pre3 = abs((VisLineA0(3) + VisLineA1(3)*preDis + VisLineA2(3)*(preDis^2) + VisLineA3(3)*(preDis^3)) - y3);
delta_d2 = abs(d_pre2 - d_cur2);
delta_d3 = abs(d_pre3 - d_cur3);

== matlab function PvtSubSys_LSM/Subsystem/TargetLineCalc_20ms/TargetLineCalc/Subsystem5/MATLAB Function7 ==
  data: dy2_Ran output; L2_R input; dy3_Ran output; L3_R input
function [dy2_Ran,dy3_Ran] = fcn(L2_R,L3_R)
dy2_Ran = L2_R;
dy3_Ran= L3_R;

== matlab function PvtSubSys_LSM/Subsystem/TargetLineCalc_20ms/TargetLineCalc/MATLAB Function5 ==
  data: LH1Wij input; LH2Wij input; LH1_Valid output; LH2_Valid output; Wij_state output; kap input; preDis input; VisLineA3 input; VisLineA2 input; VisLineA1 input; VisLineA0 input
function [LH1_Valid,LH2_Valid,Wij_state] = fcn(LH1Wij,LH2Wij,...
    kap,preDis,VisLineA3,VisLineA2,VisLineA1,VisLineA0)

LH1_Valid = false;
LH2_Valid = false;
Wij_state = uint8(0);

dy_pre = 0.5*kap*preDis^2;
Curature2_pre = VisLineA1(2) + 2*VisLineA2(2)*preDis + 3*VisLineA3(2)*(preDis^2);
Curature3_pre = VisLineA1(3) + 2*VisLineA2(3)*preDis + 3*VisLineA3(3)*(preDis^2);
dy2 = (VisLineA0(2) + VisLineA1(2)*preDis + VisLineA2(2)*(preDis^2) + VisLineA3(2)*(preDis^3) - dy_pre)/sqrt(Curature2_pre^2+single(1));
dy3 = (VisLineA0(3) + VisLineA1(3)*preDis + VisLineA2(3)*(preDis^2) + VisLineA3(3)*(preDis^3) - dy_pre)/sqrt(Curature3_pre^2+single(1));
RoadWidth_Cur = VisLineA0(2)-VisLineA0(3);

if LH1Wij >= 0.3 && LH2Wij >= 0.3  %置信度都比较高
%     if LeftLightReq
%        LH1_Valid = true;
%        Wij_state = uint8(1);
%     elseif RightLightReq  %开启右转向
%         LH2_Valid = true;
%         Wij_state = uint8(2);
%     elseif StubValid>0 && StubStartDis<60 && (Direction==3 || Direction==1)  % 导航向左
%                 LH1_Valid = true;
%                 Wij_state = uint8(3);
%     elseif StubValid>0 && StubStartDis<60 && (Direction==4 || Direction==2)  % 导航向右
%                 LH2_Valid = true;
%                 Wij_state = uint8(4);
    
    if RoadWidth_Cur-(dy2-dy3)>0.5  || dy2-dy3-RoadWidth_Cur>0.5 ||...
            abs(VisLineA0(2) - VisLineA0(3))>4.2 ||...
            abs(VisLineA0(2) - VisLineA0(3))<2.6     %没方向，有分叉或过宽、过窄
        if LH1Wij >= LH2Wij
            LH1_Valid = true;
            Wij_state = uint8(3);
        else
            LH2_Valid = true;
            Wij_state = uint8(4);
        end
    else  %没方向，没分叉
        LH1_Valid = true;
        LH2_Valid = true;
        Wij_state = uint8(5);
    end
    
elseif LH1Wij >= 0.3 
    LH1_Valid = true;
    Wij_state = uint8(1);
elseif LH2Wij >= 0.3
    LH2_Valid = true;
    Wij_state = uint8(2);
end

== matlab function PvtSubSys_LSM/Subsystem/TargetLineCalc_20ms/TargetLineCalc/MATLAB Function6 ==
  data: LeftOffset_b input boolean; RightOffset_b input boolean; LCKSts input; HWASts input; HWAStsK1 input; LaneChangeCancel_b output; LckLock_b output; Cnt1K1 input uint8; Cnt2K1 input uint8; Cnt1 output; Cnt2 output
function [LaneChangeCancel_b,LckLock_b,Cnt1,Cnt2] = ...
    fcn(LeftOffset_b,RightOffset_b,LCKSts,HWASts,HWAStsK1,Cnt1K1,Cnt2K1)

Cnt1 = max(Cnt1K1-uint8(1),uint8(0));
Cnt2 = max(Cnt2K1-uint8(1),uint8(0));

if HWASts==3 && (HWAStsK1==5||HWAStsK1==6)
    Cnt1 = uint8(250);
end

if Cnt1>0
    LaneChangeCancel_b = true;
else
    LaneChangeCancel_b = false;
end

if (LaneChangeCancel_b==false)&&...
        (HWASts~=5)&&(HWASts~=6)&&...
        (LCKSts==3)
   if LeftOffset_b || RightOffset_b
      Cnt2 = uint8(250);
   end
end

if LCKSts==1||LCKSts==0||LCKSts==2
    Cnt1 = uint8(0);
    Cnt2 = uint8(0);
end

if Cnt2>0
    LckLock_b = true;
else
    LckLock_b = false;
end

== matlab function PvtSubSys_LSM/Subsystem/TargetLineCalc_20ms/TargetLineCalc/Subsystem4/MATLAB Function2 ==
  data: HWASts input; Changelane output; HWAStsK1 input; Lock_counterK1 input uint8; Lock_counter output
function [Changelane,Lock_counter]  = fcn(HWASts,HWAStsK1,Lock_counterK1)
Lock_counter = max(Lock_counterK1-uint8(1),uint8(0));
Changelane = uint8(0);
if HWASts == 5 || HWASts == 6
    Changelane = uint8(1);
elseif HWASts==3
    if HWAStsK1==5 || HWAStsK1==6 ||HWAStsK1==1 || HWAStsK1==2
        Lock_counter = uint8(250);
    end
    if Lock_counter>0
        Changelane = uint8(1);
    end
end

== matlab function PvtSubSys_LSM/Subsystem/TargetLineCalc_20ms/TargetLineCalc/LineSelect ==
  data: TJALineValid output boolean size=1; CentLaneValid input boolean size=1; CentLineA3 input single size=1; CentLineA2 input single size=1; CentLineA1 input single size=1; CentLineA0 input single size=1; CentRange input single size=1; OTLineValid input boolean size=1; aOTL input single size=1; bOTL input single size=1; cOTL input single size=1; dOTL input single size=1; dxMax input single size=1; TJA_Line_State input; TJALineA3 output single size=1; TJALineA2 output single size=1; TJALineA1 output single size=1; TJALineA0 output single size=1; TJALineRange output single size=1; LCKLineValid output boolean size=1; LCKLineA3 output single size=1; LCKLineA2 output single size=1; LCKLineA1 output single size=1; LCKLineA0 output single size=1; LCKLineRange output single size=1
function [TJALineValid,TJALineA3,TJALineA2,TJALineA1,TJALineA0,TJALineRange,...
    LCKLineValid,LCKLineA3,LCKLineA2,LCKLineA1,LCKLineA0,LCKLineRange] = ...
    LineSelect(CentLaneValid,CentLineA3,CentLineA2,CentLineA1,CentLineA0,CentRange,...
    OTLineValid,aOTL,bOTL,cOTL,dOTL,dxMax,TJA_Line_State)

TJALineValid = false;
TJALineA3 = single(0);
TJALineA2 = single(0);
TJALineA1 = single(0);
TJALineA0 = single(0);
TJALineRange = single(0);

if (CentLaneValid==true)&&(CentRange>12)
    LCKLineValid = true;
    LCKLineA3 = CentLineA3;
    LCKLineA2 = CentLineA2;
    LCKLineA1 = CentLineA1;
    LCKLineA0 = CentLineA0;
    LCKLineRange = CentRange;
else
    LCKLineValid = false;
    LCKLineA3 = single(0);
    LCKLineA2 = single(0);
    LCKLineA1 = single(0);
    LCKLineA0 = single(0);
    LCKLineRange = single(0);
end

% TJALimitSpd = 20;
% temp = (TJALimitSpd - 1.3)/1.03;
% temp = temp/3.6;


if TJA_Line_State == 1 || TJA_Line_State == 0
   
    TJALineValid = CentLaneValid;
    TJALineA3 = CentLineA3;
    TJALineA2 = CentLineA2;
    TJALineA1 = CentLineA1;
    TJALineA0 = CentLineA0;
    TJALineRange = CentRange;
elseif TJA_Line_State == 2
    TJALineValid = OTLineValid;
    TJALineA3 = aOTL;
    TJALineA2 = bOTL;
    TJALineA1 = cOTL;
    TJALineA0 = dOTL;
    TJALineRange = dxMax;
end

== matlab function PvtSubSys_LSM/Subsystem/TargetLineCalc_20ms/TargetLineCalc/Subsystem5/MATLAB Function2 ==
  data: HWASts input; Changelane output; HWAStsK1 input; Lock_counterK1 input uint8; Lock_counter output
function [Changelane,Lock_counter]  = fcn(HWASts,HWAStsK1,Lock_counterK1)
Lock_counter = max(Lock_counterK1-uint8(1),uint8(0));
Changelane = uint8(0);
if HWASts == 5 || HWASts == 6
    Changelane = uint8(1);
elseif HWASts==3
    if HWAStsK1==5 || HWAStsK1==6 ||HWAStsK1==1 || HWAStsK1==2
        Lock_counter = uint8(250);
    end
    if Lock_counter>0
        Changelane = uint8(1);
    end
end

== matlab function PvtSubSys_LSM/Subsystem/TargetLineCalc_20ms/TargetLineCalc/Subsystem5/MATLAB Function8 ==
  data: VisLineReliable input; dy2_Rel output; dy3_Rel output
function [dy2_Rel,dy3_Rel] = fcn(VisLineReliable)
dy2_Rel = VisLineReliable(2);
dy3_Rel = VisLineReliable(3);

== matlab function PvtSubSys_LSM/Subsystem/TargetLineCalc_20ms/TargetLineCalc/Subsystem2/MATLAB Function ==
  data: TJA_Line input; DOP_CO input; DOP_C1 input; DOP_C2 input; DOP_CO_EN_Limit input; DOP_C1_EN_Limit input; DOP_C2_EN_Limit input; DOP_CO_out_Limit input; DOP_C1_out_Limit input; DOP_C2_out_Limit input; DOP_In_Pre2Dop_Dis input; DOP_Out_Pre2Dop_Dis input; DOP_Valid input; dy_pre input; Y_DOP input; DOP_In_Enable output boolean; DOP_Out_Enable output
function [DOP_In_Enable,DOP_Out_Enable] = fcn(TJA_Line,DOP_CO,DOP_C1,DOP_C2,DOP_CO_EN_Limit,DOP_C1_EN_Limit,...
    DOP_C2_EN_Limit,DOP_CO_out_Limit,DOP_C1_out_Limit,DOP_C2_out_Limit,DOP_In_Pre2Dop_Dis,DOP_Out_Pre2Dop_Dis,DOP_Valid,dy_pre,Y_DOP)
DOP_In_Enable = false;
DOP_Out_Enable = false;
if TJA_Line~=2 && DOP_Valid>0
    if abs(DOP_CO)<DOP_CO_EN_Limit&&...
            abs(DOP_C1)<DOP_C1_EN_Limit&&...
            abs(DOP_C2)<DOP_C2_EN_Limit&&...
            abs(dy_pre-Y_DOP)<DOP_In_Pre2Dop_Dis
        
        DOP_In_Enable = true;
        
    end
elseif TJA_Line==2
     if abs(DOP_CO)>DOP_CO_out_Limit||...
             abs(DOP_C1)>DOP_C1_out_Limit||...
             abs(DOP_C2)>DOP_C2_out_Limit||...
             abs(dy_pre-Y_DOP)>DOP_Out_Pre2Dop_Dis||...
             DOP_Valid==0
         
        DOP_Out_Enable = true;
        
     end
end

== stateflow chart PvtSubSys_LSM/Subsystem/TargetLineCalc_20ms/TargetLineCalc/Subsystem2/TJA_Line_Select ==
  state OFF
    en:
    TJA_Line = uint8(0);
    TJA_Source = uint8(0);
  state DOP_Line
    en:
    TJA_Line = uint8(2);
    TJA_Source = uint8(1);
  state EQ4_Line
    en:
    TJA_Line = uint8(1);
    TJA_Source = uint8(0);
  (default) -> OFF
  OFF -> DOP_Line [order 2] : [Off2DOP_flag]
  OFF -> EQ4_Line [order 1] : [Off2Cent_flag]
  DOP_Line -> OFF [order 2] : [DOP2Off_flag]
  EQ4_Line -> OFF [order 2] : [Cent2Off_flag]
  EQ4_Line -> DOP_Line [order 1] : [Cent2DOP_flag]
  DOP_Line -> EQ4_Line [order 1] : [DOP2Cent_flag]
  data: TJA_Line output uint8 size=1; Cent2Off_flag input uint8 size=1; DOP2Cent_flag input uint8 size=1; DOP2Off_flag input uint8 size=1; Off2Cent_flag input uint8 size=1; Off2DOP_flag input uint8 size=1; Cent2DOP_flag input uint8 size=1; TJA_Source output uint8 size=1

== matlab function PvtSubSys_LSM/Subsystem/TargetLineCalc_20ms/TargetLineCalc/Subsystem2/LineSelect1 ==
  data: Off2Cent_flag output; Off2DOP_flag output; Cent2Off_flag output; DOP2Off_flag output; Cent2DOP_flag output; DOP2Cent_flag output; dy_pre output; Y_DOP output; Pre_dis input single; Line_State input; kap input single size=1; LCKSts input; CentLaneValid input boolean size=1; CentLineA3 input single size=1; CentLineA2 input single size=1; CentLineA1 input single size=1; CentLineA0 input single size=1; CentRange input single size=1; aOTL input single size=1; bOTL input single size=1; cOTL input single size=1; dOTL input single size=1; VisEdgeConf input uint8; VisEdgeA3 input single size=2; VisEdgeA2 input single size=2; VisEdgeA1 input single size=2; VisEdgeA0 input single size=2; DoubleLine_Pre2Cent_Dislimit input; DoubleLine_Curr2Cent_Dislimit input; DoubleLine_Dop2Cent_Dislimit input; SingleLine_Cent2Edge_Dislimit input; SingleLine_Pre2Cent_Dislimit input; SingleLine_Curr2Cent_Dislimit input; SingleLine_Dop2Cent_Dislimit input; SingleLine_DOPOut_C1 input; DoubleLine_DOPOut_C1 input; Vehicle_Speed input; DOP_EN input boolean; DOP_OUT input boolean
function [Off2Cent_flag,Off2DOP_flag,Cent2Off_flag,DOP2Off_flag,Cent2DOP_flag,DOP2Cent_flag,dy_pre,Y_DOP]= ...
    LineSelect(Pre_dis,Line_State,kap,LCKSts,...
    CentLaneValid,CentLineA3,CentLineA2,CentLineA1,CentLineA0,CentRange,...
    aOTL,bOTL,cOTL,dOTL,...
    VisEdgeConf,VisEdgeA3,VisEdgeA2,VisEdgeA1,VisEdgeA0,...
    DoubleLine_Pre2Cent_Dislimit,DoubleLine_Curr2Cent_Dislimit,DoubleLine_Dop2Cent_Dislimit,...
    SingleLine_Cent2Edge_Dislimit,SingleLine_Pre2Cent_Dislimit,SingleLine_Curr2Cent_Dislimit,SingleLine_Dop2Cent_Dislimit,...
    SingleLine_DOPOut_C1,DoubleLine_DOPOut_C1,...
    Vehicle_Speed,DOP_EN,DOP_OUT)

DOP2Cent_flag = uint8(0);
Off2Cent_flag=uint8(0);
Off2DOP_flag=uint8(0);
Cent2Off_flag=uint8(0);
DOP2Off_flag=uint8(0);
Cent2DOP_flag=uint8(0);

dy_pre = 0.5*kap*Pre_dis^2;

% CuratureCent_pre = CentLineA1 + 2*CentLineA2*preDis + 3*CentLineA3*(preDis^2);
CuratureDop_pre = cOTL + 2*bOTL*Pre_dis + 3*aOTL*(Pre_dis^2);
Y_Line = CentLineA0+CentLineA1*Pre_dis+CentLineA2*Pre_dis^2+CentLineA3*Pre_dis^3;
Y_DOP = dOTL+cOTL*Pre_dis+bOTL*Pre_dis^2+aOTL*Pre_dis^3;
dyLeRE = (VisEdgeA0(1) + VisEdgeA1(1)*Pre_dis + VisEdgeA2(1)*(Pre_dis^2) + VisEdgeA3(1)*(Pre_dis^3) - dy_pre)/sqrt(CuratureDop_pre^2+single(1));
dyRiRE = (VisEdgeA0(2) + VisEdgeA1(2)*Pre_dis + VisEdgeA2(2)*(Pre_dis^2) + VisEdgeA3(2)*(Pre_dis^3) - dy_pre)/sqrt(CuratureDop_pre^2+single(1));

Error = Y_Line-Y_DOP;
Error2= dy_pre - Y_Line;





%%       DOP到车道线切换    
% DoubleLine_Pre2Cent_Dislimit = 1
% DoubleLine_Curr2Cent_Dislimit = 0.5
% DoubleLine_Dop2Cent_Dislimit =0.5

% SingleLine_Cent2Edge_Dislimit =100

% SingleLine_Pre2Cent_Dislimit = 0.5
% SingleLine_Curr2Cent_Dislimit = 0.2
% SingleLine_Dop2Cent_Dislimit =0.2

if DOP_OUT==1&&Line_State~=0
     DOP2Cent_flag = uint8(1);
elseif DOP_OUT==0
    if Line_State~=1 && Line_State~=2 && Line_State~=0 
        if (abs(Error2)<DoubleLine_Pre2Cent_Dislimit || abs(CentLineA0)<DoubleLine_Curr2Cent_Dislimit || abs(Error)< DoubleLine_Dop2Cent_Dislimit)&&...
                abs(CentLineA1)<DoubleLine_DOPOut_C1
            DOP2Cent_flag = uint8(1);
        end
    else
        if Line_State~=0 
%             if ((VisEdgeConf(1)>=1 && abs(abs(dyLeRE-Y_Line)-abs(VisEdgeA0(1)-CentLineA0))<SingleLine_Cent2Edge_Dislimit)||...
%                     (VisEdgeConf(2)>=1 && abs(abs(dyRiRE-Y_Line)-abs(VisEdgeA0(2)-CentLineA0))<SingleLine_Cent2Edge_Dislimit)) &&...
            if (abs(Error2)<SingleLine_Pre2Cent_Dislimit || abs(CentLineA0)<SingleLine_Curr2Cent_Dislimit || abs(Error)< SingleLine_Dop2Cent_Dislimit)&&...
                    abs(CentLineA1)<SingleLine_DOPOut_C1
                DOP2Cent_flag = uint8(1);
            end
        end

    end
end


%%       OFF到车道线
if  CentLaneValid==true
    Off2Cent_flag=uint8(1);
end
%%       OFF到DOP
if DOP_EN==1 && Vehicle_Speed<55
    Off2DOP_flag=uint8(1);
end
%%       车道线到OFF
if Line_State==0
    Cent2Off_flag=uint8(1);
end
%%       DOP到OFF
if DOP_OUT==1||Vehicle_Speed>=60
    DOP2Off_flag=uint8(1);
end
%%       车道线到DOP
if Line_State==0&&DOP_EN==1&&Vehicle_Speed<55
    Cent2DOP_flag=uint8(1);
end
